simulink model "leyesmaxwell"  (R2022b)
settings: Solver=VariableStepAuto  StartTime=0.0  StopTime=10.0  RelTol=1e-3
libraries: matrix_library x1
settings Model: Creator=gonza  LastModifiedBy=gonza

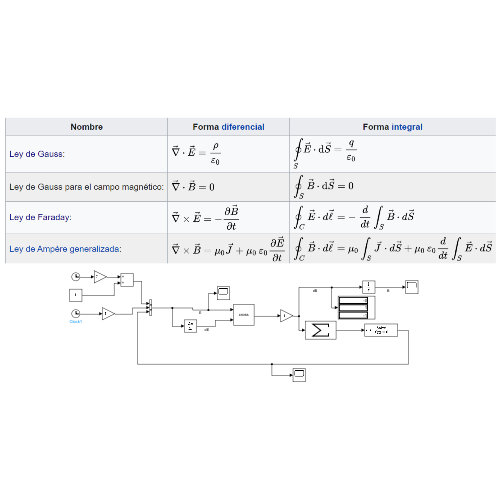
[thumbnail: Simulink's stored preview of the top-level diagram]
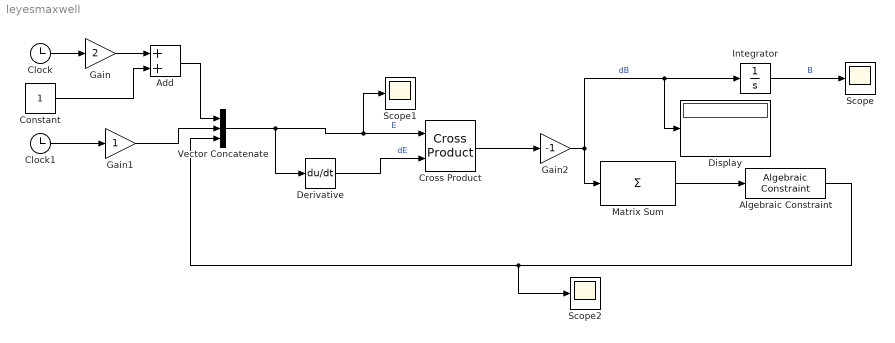
== system leyesmaxwell ==
  Add : Sum
  Algebraic Constraint : AlgebraicConstraint
  Clock : Clock
  Clock1 : Clock
  Constant : Constant
  Cross Product : matrix_library/Cross Product
  Derivative : Derivative
  Display : Display
  Gain : Gain  Gain=2
  Gain1 : Gain
  Gain2 : Gain  Gain=-1
  Integrator : Integrator  InitialCondition=[7,4,2]
  Matrix Sum : Sum  Inputs=+
  Scope : Scope
  Scope1 : Scope
  Scope2 : Scope
  Vector Concatenate : Concatenate  NumInputs=3
  wires:
  Clock/1 -> Gain/1
  Gain/1 -> Add/1
  Constant/1 -> Add/2
  Clock1/1 -> Gain1/1
  Add/1 -> Vector Concatenate/1
  Gain1/1 -> Vector Concatenate/2
  Vector Concatenate/1 -> Derivative/1, Scope1/1, Cross Product/1  "E"
  Derivative/1 -> Cross Product/2  "dE"
  Cross Product/1 -> Gain2/1
  Integrator/1 -> Scope/1  "B"
  Matrix Sum/1 -> Algebraic Constraint/1
  Algebraic Constraint/1 -> Scope2/1, Vector Concatenate/3
  Gain2/1 -> Display/1, Integrator/1, Matrix Sum/1  "dB"
